simulink model "sampleModel1451"  (R2023a)
settings: Solver=VariableStepAuto  StartTime=0.0  StopTime=10.0  RelTol=1e-3
libraries: hdlsllib x6, simulink x1
settings Model: Creator=user1  LastModifiedBy=user1

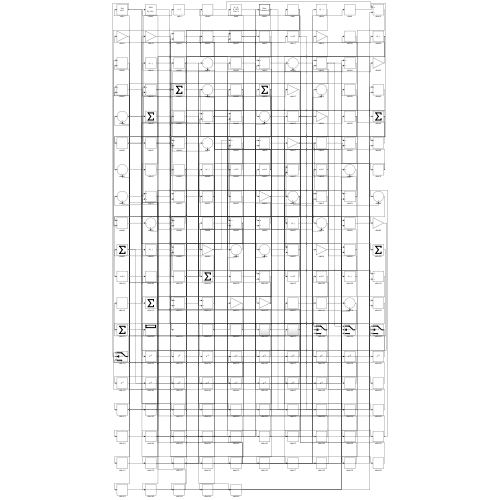
[thumbnail: Simulink's stored preview of the top-level diagram]
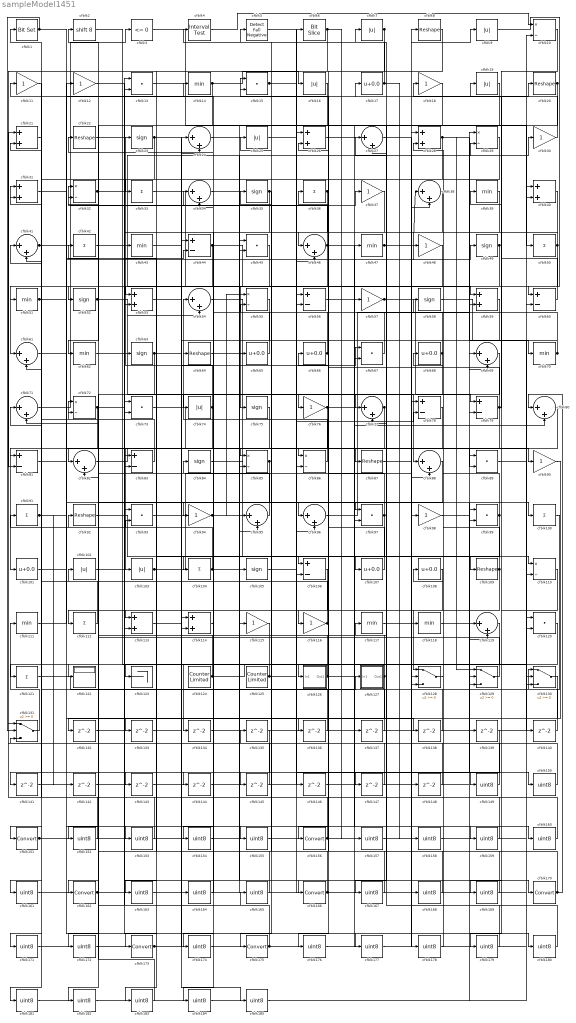
== system sampleModel1451 ==
  cfblk1 : simulink/Logic and Bit Operations/Bit Set  iBit=0
      settings: LibrarySourceBlock=|
      | hdlsllib/Logic and Bit
      | Operations/Bit Set
  cfblk{10,29,32,55,72,85..86,110} (8 alike) : Product  Inputs=*/  RndMeth=Zero  SaturateOnIntegerOverflow=on
  cfblk{33,36,42,50,91,100,104,112,121} (9 alike) : Sum  Inputs=+
  cfblk{17,65..66,68,101,107..108} (7 alike) : Bias  Bias=0.0  SaturateOnIntegerOverflow=off
  cfblk{7,9,16,19,25,74,102..103} (8 alike) : Abs  SaturateOnIntegerOverflow=off
  cfblk{23,35,49,52,58,63,75,84,105} (9 alike) : Signum
  cfblk{44,56,60,78..79,81,83,106} (8 alike) : Sum  Inputs=+-
  cfblk{8,20,22,64,87,92,109} (7 alike) : Reshape
  cfblk{11..12,18,30,37,48,57,76,90,94,98,115..116} (13 alike) : Gain
  cfblk{14,39,43,47,51,62,70,111,117..118} (10 alike) : MinMax
  cfblk{21,26,28,31,40,53,59,113..114} (9 alike) : Sum
  cfblk{24,27,34,38,41,46,54,61,69,71,77,80,82,88,95..96,119} (17 alike) : Sum  Inputs=|++
  cfblk{13,15,45,67,73,89,93,97,99,120} (10 alike) : DotProduct  OutDataTypeStr=Inherit: Inherit via internal rule
  cfblk122 : Display
  cfblk123 : Terminator
  cfblk124 : hdlsllib/Sources/Counter Limited  uplimit=7  tsamp=-1
  cfblk125 : hdlsllib/Sources/Counter Limited  uplimit=7  tsamp=-1
  cfblk126 : Subsystem
      settings: LibrarySourceBlock=|
      | hdlsllib/Ports &
      | Subsystems/Subsystem
  cfblk127 : Subsystem
      settings: LibrarySourceBlock=|
      | hdlsllib/Ports &
      | Subsystems/Subsystem
  cfblk{128..131} (4 alike) : Switch  SaturateOnIntegerOverflow=off  InputSameDT=off
  cfblk{132..148} (17 alike) : Delay  SampleTime=1
  cfblk{149..150,152..155,157..161,163..165,167..169,171..172,174,176..185} (30 alike) : DataTypeConversion  OutDataTypeStr=uint8  SaturateOnIntegerOverflow=off  RndMeth=Floor
  cfblk{151,156,162,166,170,173,175} (7 alike) : DataTypeConversion  SaturateOnIntegerOverflow=off  RndMeth=Floor
  cfblk2 : ArithShift  BitShiftNumber=8
  cfblk3 : hdlsllib/Logic and Bit Operations/Compare To Zero  relop=<=  OutDataTypeStr=boolean
  cfblk4 : hdlsllib/Logic and Bit Operations/Interval Test  IntervalClosedRight=on  uplimit=0.5  IntervalClosedLeft=on  lowlimit=-0.5  OutDataTypeStr=boolean
  cfblk5 : hdlsllib/Logic and Bit Operations/Detect Fall Negative  vinit=0  OutDataTypeStr=boolean
  cfblk6 : hdlsllib/Logic and Bit Operations/Bit Slice  lidx=7  ridx=0
  wires:
  cfblk2/1 -> cfblk126/1(In1)
  cfblk47/1 -> cfblk38/1, cfblk88/2, cfblk148/1
  cfblk44/1 -> cfblk59/1, cfblk51/1, cfblk29/2
  cfblk82/1 -> cfblk90/1
  cfblk86/1 -> cfblk54/1
  cfblk131/1 -> cfblk111/1
  cfblk30/1 -> cfblk18/1
  cfblk104/1 -> cfblk105/1, cfblk91/1
  cfblk115/1 -> cfblk162/1
  cfblk9/1 -> cfblk60/1
  cfblk35/1 -> cfblk145/1, cfblk163/1
  cfblk42/1 -> cfblk166/1
  cfblk71/1 -> cfblk37/1
  cfblk85/1 -> cfblk103/1, cfblk182/1
  cfblk40/1 -> cfblk156/1
  cfblk8/1 -> cfblk173/1
  cfblk92/1 -> cfblk107/1
  cfblk74/1 -> cfblk93/1, cfblk63/1
  cfblk96/1 -> cfblk29/1
  cfblk26/1 -> cfblk110/1
  cfblk72/1 -> cfblk101/1, cfblk48/1
  cfblk63/1 -> cfblk129/2, cfblk152/1
  cfblk48/1 -> cfblk61/1
  cfblk64/1 -> cfblk100/1
  cfblk33/1 -> cfblk75/1
  cfblk41/1 -> cfblk3/1, cfblk177/1
  cfblk73/1 -> cfblk86/1
  cfblk70/1 -> cfblk25/1, cfblk65/1
  cfblk95/1 -> cfblk71/2
  cfblk23/1 -> cfblk114/1, cfblk161/1
  cfblk57/1 -> cfblk79/1, cfblk109/1
  cfblk24/1 -> cfblk170/1
  cfblk76/1 -> cfblk99/2, cfblk171/1
  cfblk54/1 -> cfblk88/1
  cfblk84/1 -> cfblk120/1
  cfblk14/1 -> cfblk16/1, cfblk33/1
  cfblk38/1 -> cfblk76/1
  cfblk87/1 -> cfblk78/1
  cfblk3/1 -> cfblk95/1
  cfblk77/1 -> cfblk106/1, cfblk85/2
  cfblk121/1 -> cfblk127/1(In1)
  cfblk62/1 -> cfblk23/1
  cfblk102/1 -> cfblk13/2
  cfblk20/1 -> cfblk97/2, cfblk147/1
  cfblk112/1 -> cfblk31/1
  cfblk15/1 -> cfblk26/1, cfblk89/2
  cfblk65/1 -> cfblk22/1
  cfblk66/1 -> cfblk15/1, cfblk34/1
  cfblk105/1 -> cfblk78/2
  cfblk128/1 -> cfblk58/1
  cfblk103/1 -> cfblk44/1, cfblk9/1
  cfblk19/1 -> cfblk62/1
  cfblk34/1 -> cfblk86/2
  cfblk21/1 -> cfblk151/1
  cfblk107/1 -> cfblk15/2
  cfblk32/1 -> cfblk30/1, cfblk118/1
  cfblk119/1 -> cfblk175/1
  cfblk113/1 -> cfblk67/1
  cfblk116/1 -> cfblk112/1, cfblk61/2
  cfblk124/1 -> cfblk2/1, cfblk128/2
  cfblk37/1 -> cfblk74/1
  cfblk78/1 -> cfblk82/1
  cfblk111/1 -> cfblk17/1
  cfblk79/1 -> cfblk26/2, cfblk97/1, cfblk39/1
  cfblk50/1 -> cfblk87/1, cfblk46/1, cfblk77/2
  cfblk7/1 -> cfblk116/1, cfblk143/1
  cfblk75/1 -> cfblk81/1
  cfblk22/1 -> cfblk20/1
  cfblk100/1 -> cfblk130/1
  cfblk18/1 -> cfblk52/1
  cfblk125/1 -> cfblk121/1, cfblk130/2
  cfblk52/1 -> cfblk54/2, cfblk77/1
  cfblk28/1 -> cfblk123/1, cfblk70/1, cfblk129/1
  cfblk58/1 -> cfblk120/2
  cfblk91/1 -> cfblk49/1, cfblk142/1
  cfblk13/1 -> cfblk50/1
  cfblk80/1 -> cfblk83/1
  cfblk93/1 -> cfblk47/1
  cfblk60/1 -> cfblk19/1
  cfblk94/1 -> cfblk67/2, cfblk55/1
  cfblk101/1 -> cfblk44/2
  cfblk46/1 -> cfblk32/1, cfblk104/1, cfblk129/3
  cfblk59/1 -> cfblk114/2
  cfblk114/1 -> cfblk64/1
  cfblk36/1 -> cfblk53/2, cfblk144/1
  cfblk51/1 -> cfblk12/1, cfblk153/1
  cfblk129/1 -> cfblk72/1
  cfblk29/1 -> cfblk73/2
  cfblk49/1 -> cfblk106/2, cfblk141/1
  cfblk12/1 -> cfblk96/1
  cfblk127/1(Out1) -> cfblk34/2, cfblk172/1
  cfblk118/1 -> cfblk89/1
  cfblk99/1 -> cfblk55/2, cfblk176/1
  cfblk126/1(Out1) -> cfblk32/2, cfblk80/2
  cfblk97/1 -> cfblk113/1, cfblk36/1
  cfblk108/1 -> cfblk128/1
  cfblk83/1 -> cfblk31/2
  cfblk16/1 -> cfblk53/1
  cfblk61/1 -> cfblk85/1
  cfblk67/1 -> cfblk14/1
  cfblk1/1 -> cfblk131/2, cfblk96/2, cfblk94/1
  cfblk68/1 -> cfblk11/1, cfblk82/2
  cfblk6/1 -> cfblk81/2, cfblk157/1
  cfblk106/1 -> cfblk113/2
  cfblk4/1 -> cfblk10/1
  cfblk17/1 -> cfblk4/1, cfblk158/1
  cfblk11/1 -> cfblk41/2
  cfblk109/1 -> cfblk122/1, cfblk28/2
  cfblk90/1 -> cfblk132/1
  cfblk88/1 -> cfblk133/1
  cfblk120/1 -> cfblk134/1
  cfblk134/1 -> cfblk110/2
  cfblk130/1 -> cfblk136/1
  cfblk136/1 -> cfblk93/2
  cfblk137/1 -> cfblk41/1
  cfblk31/1 -> cfblk138/1
  cfblk138/1 -> cfblk71/1
  cfblk89/1 -> cfblk140/1
  cfblk140/1 -> cfblk13/1
  cfblk141/1 -> cfblk38/2
  cfblk142/1 -> cfblk46/2
  cfblk143/1 -> cfblk95/2
  cfblk144/1 -> cfblk79/2
  cfblk145/1 -> cfblk1/1
  cfblk25/1 -> cfblk146/1
  cfblk146/1 -> cfblk99/1
  cfblk147/1 -> cfblk131/1
  cfblk148/1 -> cfblk131/3
  cfblk5/1 -> cfblk149/1
  cfblk149/1 -> cfblk7/1
  cfblk98/1 -> cfblk150/1
  cfblk150/1 -> cfblk5/1
  cfblk151/1 -> cfblk137/1, cfblk59/2, cfblk83/2
  cfblk152/1 -> cfblk21/1
  cfblk153/1 -> cfblk21/2
  cfblk135/1 -> cfblk154/1
  cfblk154/1 -> cfblk45/2
  cfblk81/1 -> cfblk155/1
  cfblk155/1 -> cfblk135/1
  cfblk156/1 -> cfblk28/1, cfblk92/1
  cfblk157/1 -> cfblk40/1
  cfblk158/1 -> cfblk40/2
  cfblk56/1 -> cfblk159/1
  cfblk159/1 -> cfblk108/1
  cfblk53/1 -> cfblk160/1
  cfblk160/1 -> cfblk56/1
  cfblk161/1 -> cfblk56/2
  cfblk162/1 -> cfblk128/3, cfblk6/1
  cfblk163/1 -> cfblk115/1
  cfblk43/1 -> cfblk164/1
  cfblk164/1 -> cfblk84/1
  cfblk165/1 -> cfblk43/1
  cfblk166/1 -> cfblk130/3, cfblk35/1
  cfblk39/1 -> cfblk167/1
  cfblk167/1 -> cfblk42/1
  cfblk117/1 -> cfblk168/1
  cfblk168/1 -> cfblk45/1
  cfblk110/1 -> cfblk169/1
  cfblk169/1 -> cfblk117/1
  cfblk170/1 -> cfblk80/1, cfblk66/1
  cfblk171/1 -> cfblk24/1
  cfblk172/1 -> cfblk24/2
  cfblk173/1 -> cfblk60/2, cfblk57/1
  cfblk55/1 -> cfblk174/1
  cfblk174/1 -> cfblk8/1
  cfblk175/1 -> cfblk165/1, cfblk98/1, cfblk72/2, cfblk73/1
  cfblk176/1 -> cfblk119/1
  cfblk177/1 -> cfblk119/2
  cfblk27/1 -> cfblk178/1
  cfblk178/1 -> cfblk68/1
  cfblk10/1 -> cfblk179/1
  cfblk179/1 -> cfblk27/1
  cfblk132/1 -> cfblk180/1
  cfblk180/1 -> cfblk27/2
  cfblk139/1 -> cfblk181/1
  cfblk181/1 -> cfblk10/2
  cfblk182/1 -> cfblk139/1
  cfblk69/1 -> cfblk183/1
  cfblk183/1 -> cfblk102/1
  cfblk45/1 -> cfblk184/1
  cfblk184/1 -> cfblk69/1
  cfblk133/1 -> cfblk185/1
  cfblk185/1 -> cfblk69/2

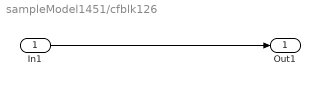
== system sampleModel1451/cfblk126 ==
  In1 : Inport
  Out1 : Outport
  wires:
  In1/1 -> Out1/1

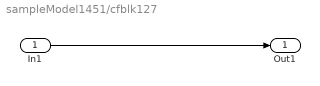
== system sampleModel1451/cfblk127 ==
  In1 : Inport
  Out1 : Outport
  wires:
  In1/1 -> Out1/1
